simulink model "integrator_test2"  (Simulink 6.1)
settings: Solver=FixedStepDiscrete  StartTime=0.0  StopTime=1000  RelTol=1e-3
undefined symbols (not defined in the file or in its folder): DiscIntNeverNeededParam
libraries: dspsigops x2, simulink x1
settings Model: Creator=svenhoffmann  LastModifiedBy=svenhoffmann  ExtModeAutoUpdateStatusClock=off
settings DataIOCC: MaxDataPoints=10000  SaveFormat=StructureWithTime
settings DebuggingCC: SolverPrmCheckMsg=warning

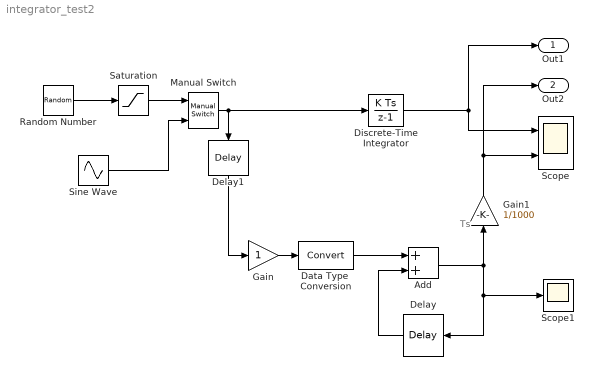
== system integrator_test2 ==
  note: Ts
  Add : Sum  OutDataTypeMode=Specify via dialog  OutDataType=sfix(32)  OutScaling=2^-14
  Data Type  Conversion : DataTypeConversion  OutDataTypeMode=Specify via dialog  OutScaling=2^-14  SaturateOnIntegerOverflow=on  RndMeth=Zero
  Delay : dspsigops/Delay  Orientation=left  dly_unit=Samples  delay=1  ic_detail=off  dif_ic_for_ch=off  dif_ic_for_dly=off  ic=0  reset_popup=None
  Delay1 : dspsigops/Delay  Orientation=down  dly_unit=Samples  delay=1  ic_detail=off  dif_ic_for_ch=off  dif_ic_for_dly=off  ic=0  reset_popup=None
  Discrete-Time Integrator : DiscreteIntegrator  SampleTime=1/1000  ICPrevOutput=DiscIntNeverNeededParam  ICPrevScaledInput=DiscIntNeverNeededParam
  Gain : Gain
  Gain1 : Gain  Orientation=up  Gain=1/1000  OutDataTypeMode=Specify via dialog  OutScaling=2^-12
  Manual Switch : simulink/Signal Routing/Manual Switch  sw=0  action=0
  Random Number : RandomNumber  Seed=3579  SampleTime=1/1000
  Saturation : Saturate  UpperLimit=1  LowerLimit=-1
  Scope : Scope  NumInputPorts=2
      settings: YMin=-0.0025~-0.0175  YMax=0.0325~0.0325
  Scope1 : Scope
      settings: YMin=-50  YMax=325
  Sine Wave : Sin  Frequency=2*pi*10  SampleTime=1/1000
  Out1 : Outport
  Out2 : Outport  Port=2
  wires:
  Delay/1 -> Add/2
  Gain/1 -> Data Type  Conversion/1
  Add/1 -> Gain1/1, Delay/1, Scope1/1
  Discrete-Time Integrator/1 -> Scope/1, Out1/1
  Data Type  Conversion/1 -> Add/1
  Random Number/1 -> Saturation/1
  Manual Switch/1 -> Discrete-Time Integrator/1, Delay1/1
  Sine Wave/1 -> Manual Switch/2
  Delay1/1 -> Gain/1
  Gain1/1 -> Scope/2, Out2/1
  Saturation/1 -> Manual Switch/1
